simulink model "MVP_NN_Control_R3"  (R2014a)
settings: Solver=ode45  StartTime=0.0  StopTime=10.0  RelTol=1e-3
undefined symbols (not defined in the file): den, num
libraries: neural x1
settings Model: Creator=david78k  LastModifiedBy=david78k

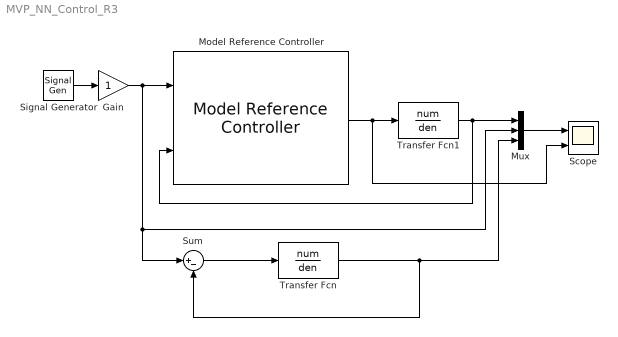
== system MVP_NN_Control_R3 ==
  Gain : Gain
  Model Reference Controller : neural/Control Systems/Model Reference Controller  Nrc=[]  Nic=[]  Njc=[]  IW_y=[]  IW_u=[]  IW_r=[]  B1_c=[]  B2_c=[]  LW_c=[]  retraining_c=[]  max_i_int=[]  min_i_int=[]  max_r_int=[]  min_r_int=[]  Ts=[]  S1=[]  Ni=[]  Nj=[]  sim_file=0  trainfun=trainlm  Use_validation=[]  Use_Testing=[]  Use_Inc_training=[]  Use_previous_weights=[]  max_i=[]  min_i=[]  max_r=[]  min_r=[]  sam_training=[]  sam_training_c=[]  epochs=[]  epochs_c=[]  minp=[]  maxp=[]  mint=[]  maxt=[]  Normalize=[]  IW=[]  LW1_2=[]  LW2_1=[]  B1=[]  B2=[]  S1c=[]  Limit_output=[]  min_output=[]  max_output=[]  Ref_file=0
  Mux : Mux  Inputs=3
  Scope : Scope  NumInputPorts=2
      settings: YMin=-5~-5  YMax=5~5
  Signal Generator : SignalGenerator  Units=rad/sec
  Sum : Sum  Inputs=|+-
  Transfer Fcn : TransferFcn  Numerator=num  Denominator=den  ContinuousStateAttributes='theta'
  Transfer Fcn1 : TransferFcn  Numerator=num  Denominator=den  ContinuousStateAttributes='theta'
  wires:
  Gain/1 -> Sum/1, Mux/2, Model Reference Controller/1
  Transfer Fcn/1 -> Mux/3, Sum/2
  Sum/1 -> Transfer Fcn/1
  Transfer Fcn1/1 -> Mux/1, Model Reference Controller/2
  Mux/1 -> Scope/1
  Signal Generator/1 -> Gain/1
  Model Reference Controller/1 -> Scope/2, Transfer Fcn1/1
